simulink model "Park"  (R2022b)
settings: Solver=ode1  StartTime=0.0  StopTime=1  FixedStep=1e-4  RelTol=1e-6  AbsTol=1e-6
PostLoadFcn:
  | , if any(exist('dsrtsu_mdlpostloadfcn', 'file') == [2, 3, 6]), try dsrtsu_mdlpostloadfcn('Execute', bdroot); catch fprintf('Error in PostLoadFcn (dsrtsu_mdlpostloadfcn) for model "%s":\n %s\n', bdroot, lasterr); end, end,
Description:
  | Standard RTI1104 template.
  | Supported MATLAB version:  R2017b.
settings Model: Tag=RTI1104  DSRTSU_INTERNAL_RTI_VER=510  DSRTSU_INTERNAL_RTI_TYPE=rti1104  RTICANMMDATA=struct('GeneralSetupData',struct('modelroot',['C:\Users\habayah\Desktop\TER MERCIER'],'generalsettings',struct('filesettings',struct('destfolder',struct('Name','RTICANMM_FILES','Check',1),'buildfolder',struct('Name','.','Check',1),'AbsDestfolder',struct('Name',['C:\Users\habayah\Desktop\TER MERCIER\RTICANMM_FILES']),'AbsBuildfolder',struct('Name',['C:\Users\habayah\Desktop\TER MERCIER']))),'options',struct('addpaths',1,'rmpaths',1,'addtrcexclusion',logical(1),'cannavigator',struct('checkmonitoring',0),'show_usrtrc',0,'use_usrtrc',0),'advanced',struct('options',[1 1 1 1 1 1 1 1 1 1 1 1 1 1 1 1 1 1 1 1 1 1 1 1 1 1 1 1 1 1 1 1 1 1 1 1 1 1 1 1 1 1 1 1 1 1 1 1 1 1 1 1 1 1 1 1 1 1 1 1 1 1 1 1 1 1 1 1 1 1 1 1 1 1 1 1 1 1 1 1 1 1 1 1 1 1 1 1 1 1 1 1 1 1 1 1 1 1 1 1]),'MPSetup',{{}},'modelname','Park','block','Park'))  DSRTSU_INTERNAL_RTIFLEXRAYCONFIG=110  DSRTSU_INTERNAL_RTIFPGA=110  Creator=habayah  LastModifiedBy=ZinouAb
settings SolverCC: AlgebraicLoopSolver=TrustRegion
settings DataIOCC: ReturnWorkspaceOutputs=off
settings OptimizationCC: BlockReduction=off  OptimizeBlockIOStorage=off  BufferReuse=off  GlobalBufferReuse=off  ExpressionFolding=off  LocalBlockOutputs=off
settings DebuggingCC: UnconnectedInputMsg=warning  UnconnectedOutputMsg=warning  UnconnectedLineMsg=warning  SFMachineParentedDataDiag=warning  ArithmeticOperatorsInVariantConditions=warning
settings HardwareCC: ProdBitPerPointer=32  ProdBitPerSizeT=32  ProdBitPerPtrDiffT=32  ProdLargestAtomicInteger=Integer  ProdEndianess=BigEndian  ProdWordSize=32  ProdHWDeviceType=Custom Processor->Custom  TargetIntDivRoundTo=Zero  TargetEndianess=BigEndian  TargetHWDeviceType=Custom Processor->Custom
settings ModelReferenceCC: EnableRefExpFcnMdlSchedulingChecks=on
settings SFSimCC: SimUseLocalCustomCode=off  MATLABDynamicMemAlloc=off  CustomCodeUndefinedFunction=UseInterfaceOnly
settings RTWCC: Description=dSPACE DS1104 Hardware Platform  SystemTargetFile=rti1104.tlc  MakeCommand=make_rti  TemplateMakefile=rti1104.tmf  RTWUseLocalCustomCode=off
settings CodeAppCC: StateflowObjectComments=on
settings STFCustomTargetCC: MatFileLogging=on  SystemTargetFile=rti1104.tlc
settings GRTTargetCC: TargetLangStandard=C89/C90 (ANSI)  ParMdlRefBuildCompliant=off  CompOptLevelCompliant=off  ConcurrentExecutionCompliant=off  CombineOutputUpdateFcns=off  CPPClassGenCompliant=off  UseToolchainInfoCompliant=off
settings ConfigComp: CovMetricSettings=dswe

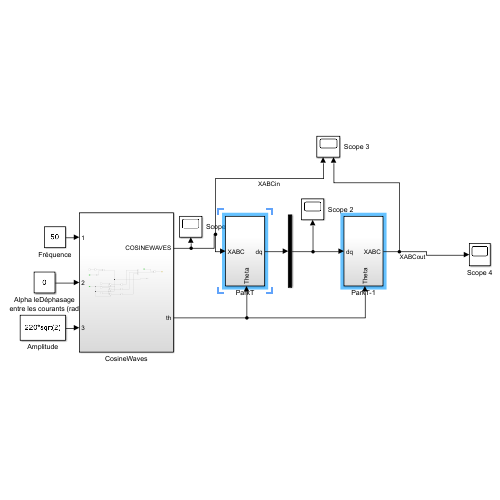
[thumbnail: Simulink's stored preview of the top-level diagram]
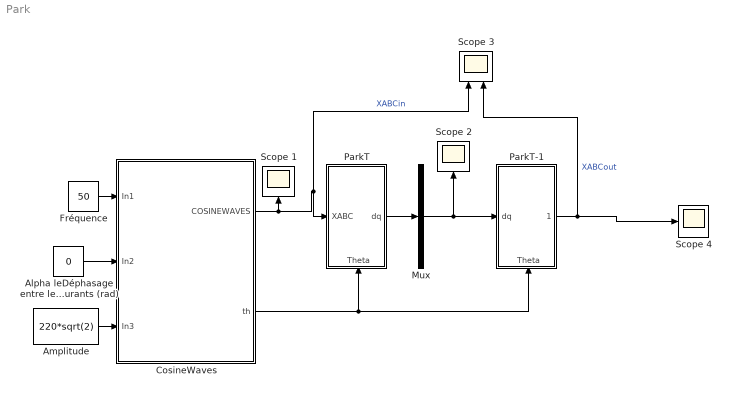
== system Park ==
  Alpha leDéphasage entre les courants (rad) : Constant  Value=0
  Amplitude : Constant  Value=220*sqrt(2)
  CosineWaves : Subsystem
  Fréquence : Constant  Value=50
  Mux : Mux  Inputs=1
  ParkT : Subsystem
      settings: PortSchema="{\"entries\":[{\"content\":{\"sides\":[{\"content\":{\"connectorIds\":[\"In1\"]},\"type\":\"ConnectorPlacement.EquallySpacedRectSide\",\"uuid\":\"228dfcfc-5d6b-4d2b-a954-ee5f3fee8856\"},{\"content\":{\"connectorIds\":[\"Out1\"],\"side\":\"RIGHT\"},\"type\":\"ConnectorPlacement.EquallySpacedRectSide\",\"uuid\":\"1b1b4c30-bceb-4aa5-9a3a-183aa9b64903\"},{\"content\":{\"connectorIds\":[],\"side\":\"TOP\"},\"type\":\"ConnectorPlacement.EquallySpacedRectSide\",\"uuid\":\"f7d3bddd-1df8-4cd8-ab8f-9e5cd0980ffa\"},{\"content\":{\"connectorIds\":[\"In2\"],\"side\":\"BOTTOM\"},\"type\":\"ConnectorPlacement.EquallySpacedRectSide\",\"uuid\":\"ca51e6a4-16df-4fde-8b7d-f74278a3171d\"}]},\"type\":\"ConnectorPlacement.EquallySpacedConnector\",\"uuid\":\"a8efb2f9-24b2-4419-8f97-2809a6aaa24c\"}],\"packageUris\":[\"http://schema.mathworks.com/mf0/Connector/R2020b\"],\"version\":\"1.0\"}"
  ParkT-1 : Subsystem
      settings: PortSchema="{\"entries\":[{\"content\":{\"sides\":[{\"content\":{\"connectorIds\":[\"In1\"]},\"type\":\"ConnectorPlacement.EquallySpacedRectSide\",\"uuid\":\"ed5ee07b-b316-480c-b9ec-652acf4aaee1\"},{\"content\":{\"connectorIds\":[\"Out1\"],\"side\":\"RIGHT\"},\"type\":\"ConnectorPlacement.EquallySpacedRectSide\",\"uuid\":\"52d50e66-916b-4a4a-9cee-3d7b4015ccc4\"},{\"content\":{\"connectorIds\":[],\"side\":\"TOP\"},\"type\":\"ConnectorPlacement.EquallySpacedRectSide\",\"uuid\":\"08f86e0e-d4d6-4b18-9159-89a705b15501\"},{\"content\":{\"connectorIds\":[\"In2\"],\"side\":\"BOTTOM\"},\"type\":\"ConnectorPlacement.EquallySpacedRectSide\",\"uuid\":\"c8ae1c02-6dab-4f60-b9b6-1b5db27b47ec\"}]},\"type\":\"ConnectorPlacement.EquallySpacedConnector\",\"uuid\":\"6fabca93-26c3-4fea-833e-475510973df7\"}],\"packageUris\":[\"http://schema.mathworks.com/mf0/Connector/R2020b\"],\"version\":\"1.0\"}"
  Scope 1 : Scope
  Scope 2 : Scope
  Scope 3 : Scope  NumInputPorts=2
  Scope 4 : Scope
  wires:
  Fréquence/1 -> CosineWaves/1(In1)
  Alpha leDéphasage entre les courants (rad)/1 -> CosineWaves/2(In2)
  CosineWaves/2(th) -> ParkT-1/2(Theta), ParkT/2(Theta)
  Mux/1 -> Scope 2/1, ParkT-1/1(dq)
  CosineWaves/1(COSINEWAVES) -> ParkT/1(XABC), Scope 3/1, Scope 1/1  "XABCin"
  Amplitude/1 -> CosineWaves/3(In3)
  ParkT/1(dq) -> Mux/1
  ParkT-1/1(XABC) -> Scope 3/2, Scope 4/1  "XABCout"

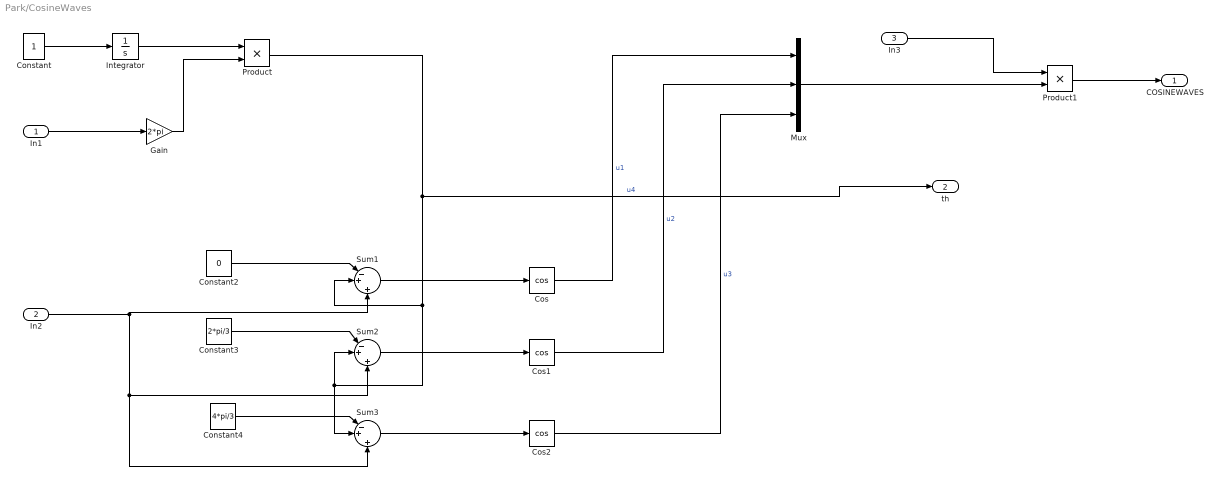
== system Park/CosineWaves ==
  In1 : Inport
  In2 : Inport  Port=2
  In3 : Inport  Port=3
  Constant : Constant
  Constant2 : Constant  Value=0
  Constant3 : Constant  Value=2*pi/3
  Constant4 : Constant  Value=4*pi/3
  Cos : Trigonometry  Operator=cos
  Cos1 : Trigonometry  Operator=cos
  Cos2 : Trigonometry  Operator=cos
  Gain : Gain  Gain=2*pi
  Integrator : Integrator
  Mux : Mux  Inputs=3
  Product : Product
  Product1 : Product
  Sum1 : Sum  Inputs=|-+|+
  Sum2 : Sum  Inputs=|-+|+
  Sum3 : Sum  Inputs=|-+|+
  COSINEWAVES : Outport
  th : Outport  Port=2
  wires:
  Constant/1 -> Integrator/1
  Sum2/1 -> Cos1/1
  In2/1 -> Sum1/3, Sum3/3, Sum2/3
  Product/1 -> th/1, Sum3/2, Sum2/2, Sum1/2  "u4"
  Constant3/1 -> Sum2/1
  Sum3/1 -> Cos2/1
  Sum1/1 -> Cos/1
  Constant2/1 -> Sum1/1
  Constant4/1 -> Sum3/1
  Gain/1 -> Product/2
  Integrator/1 -> Product/1
  In1/1 -> Gain/1
  Cos1/1 -> Mux/2  "u2"
  Cos/1 -> Mux/1  "u1"
  Cos2/1 -> Mux/3  "u3"
  Mux/1 -> Product1/2
  In3/1 -> Product1/1
  Product1/1 -> COSINEWAVES/1

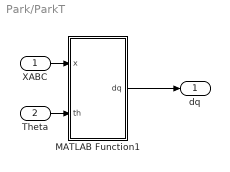
== system Park/ParkT ==
  XABC : Inport
  Theta : Inport  Port=2
  MATLAB Function1 : MATLAB Function  TreatAsAtomicUnit=on
  dq : Outport
  wires:
  Theta/1 -> MATLAB Function1/2(th)
  MATLAB Function1/1(dq) -> dq/1
  XABC/1 -> MATLAB Function1/1(x)

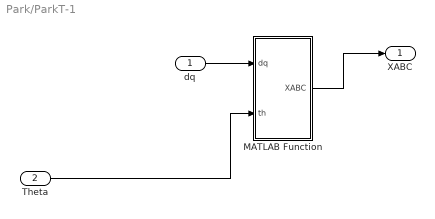
== system Park/ParkT-1 ==
  dq : Inport
  Theta : Inport  Port=2
  MATLAB Function : MATLAB Function  TreatAsAtomicUnit=on
  XABC : Outport
  wires:
  MATLAB Function/1(XABC) -> XABC/1
  dq/1 -> MATLAB Function/1(dq)
  Theta/1 -> MATLAB Function/2(th)

== matlab function Park/ParkT/MATLAB Function1 ==
  data: x input; dq output; th input
function dq = Park(x,th)
% vd=(2/3)*(u1*cos(th)+u2*cos(th-2*pi/3)+u3*cos(th+2*pi/3));
% vq=(2/3)*(-u1*sin(th)-u2*sin(th-2*pi/3)-u3*sin(th+2*pi/3));
P=(2/3)*[ cos(th) cos(th-2*pi/3) cos(th+2*pi/3);
         -sin(th) -sin(th-2*pi/3) -sin(th+2*pi/3)  ];
dq=P*x;
% xd=prod(1);
% xq=prod(2);

== matlab function Park/ParkT-1/MATLAB Function ==
  data: dq input; XABC output; th input
function XABC= Parkinv(dq,th)

parkinv = [ cos(th),           -sin(th); 
          cos(th-2*pi/3), -sin(th-2*pi/3); 
          cos(th+2*pi/3), -sin(th+2*pi/3)];

XABC = parkinv * [dq];

% x1=temp(1);
% x2=temp(2);
% x3=temp(3);
